simulink subsystem "soccer_ball_sub"  (R2022b)
settings: Solver=VariableStepAuto  StartTime=0.0  StopTime=10.0  RelTol=1e-3
settings Model: Creator=User  LastModifiedBy=ROG

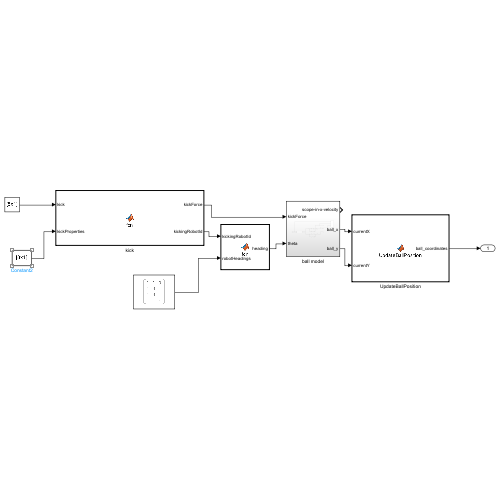
[thumbnail: Simulink's stored preview of the top-level diagram]
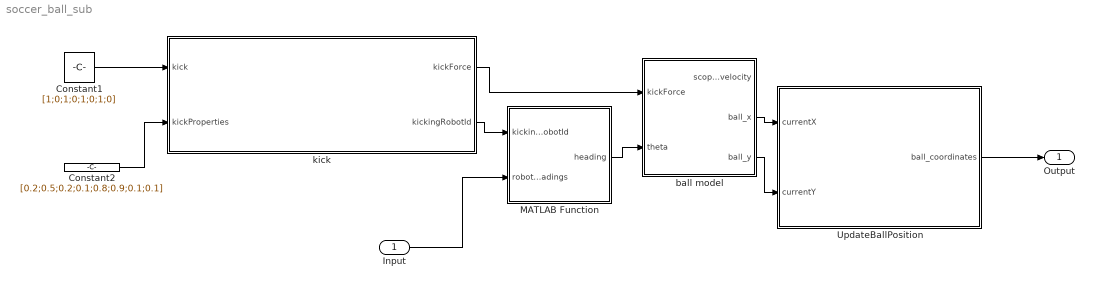
== system soccer_ball_sub ==
  Input : Inport
  Constant1 : Constant  Value=[1;0;1;0;1;0;1;0]
  Constant2 : Constant  Value=[0.2;0.5;0.2;0.1;0.8;0.9;0.1;0.1]
  MATLAB Function : MATLAB Function  TreatAsAtomicUnit=on
  UpdateBallPosition : MATLAB Function  TreatAsAtomicUnit=on
  ball model : Subsystem
  kick : MATLAB Function  TreatAsAtomicUnit=on
  Output : Outport
  wires:
  ball model/2(ball_x) -> UpdateBallPosition/1(currentX)
  kick/1(kickForce) -> ball model/1(kickForce)
  MATLAB Function/1(heading) -> ball model/2(theta)
  ball model/3(ball_y) -> UpdateBallPosition/2(currentY)
  UpdateBallPosition/1(ball_coordinates) -> Output/1
  kick/2(kickingRobotId) -> MATLAB Function/1(kickingRobotId)
  Input/1 -> MATLAB Function/2(robotHeadings)
  Constant1/1 -> kick/1(kick)
  Constant2/1 -> kick/2(kickProperties)

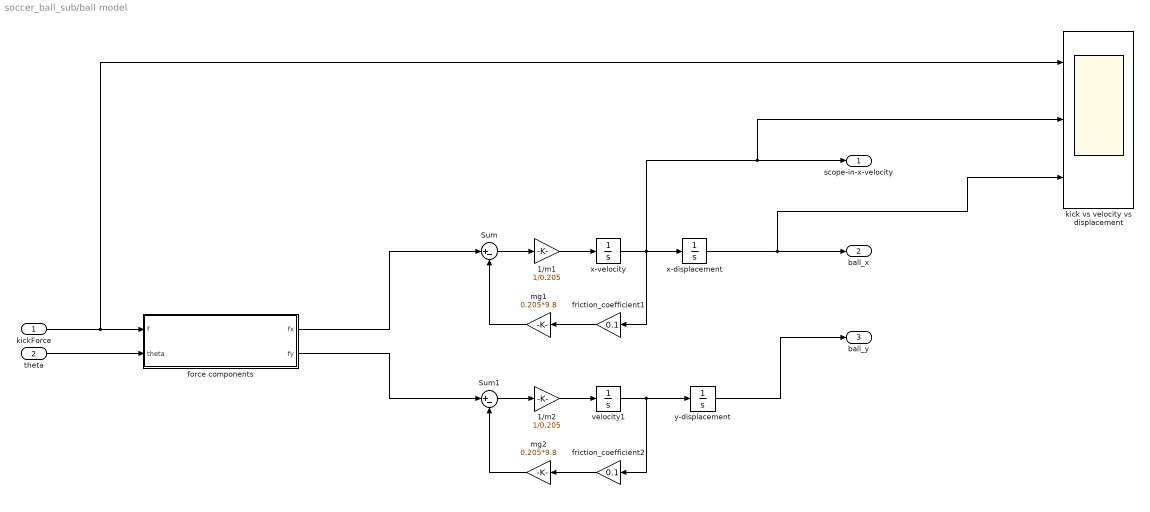
== system soccer_ball_sub/ball model ==
  kickForce : Inport
  theta : Inport  Port=2
  1/m1 : Gain  Gain=1/0.205
  1/m2 : Gain  Gain=1/0.205
  Sum : Sum  Inputs=|+-
  Sum1 : Sum  Inputs=|+-
  force components : MATLAB Function  TreatAsAtomicUnit=on
  friction_coefficient1 : Gain  Gain=0.1
  friction_coefficient2 : Gain  Gain=0.1
  kick vs velocity vs displacement : Scope  NumInputPorts=3
  mg1 : Gain  Gain=0.205*9.8
  mg2 : Gain  Gain=0.205*9.8
  velocity1 : Integrator
  x-displacement : Integrator
  x-velocity : Integrator
  y-displacement : Integrator
  scope-in-x-velocity : Outport
  ball_x : Outport  Port=2
  ball_y : Outport  Port=3
  wires:
  kickForce/1 -> force components/1(f), kick vs velocity vs displacement/1
  y-displacement/1 -> ball_y/1
  theta/1 -> force components/2(theta)
  x-displacement/1 -> ball_x/1, kick vs velocity vs displacement/3
  mg2/1 -> Sum1/2
  force components/1(fx) -> Sum/1
  1/m1/1 -> x-velocity/1
  Sum1/1 -> 1/m2/1
  force components/2(fy) -> Sum1/1
  friction_coefficient1/1 -> mg1/1
  1/m2/1 -> velocity1/1
  Sum/1 -> 1/m1/1
  mg1/1 -> Sum/2
  friction_coefficient2/1 -> mg2/1
  x-velocity/1 -> x-displacement/1, friction_coefficient1/1, scope-in-x-velocity/1, kick vs velocity vs displacement/2
  velocity1/1 -> y-displacement/1, friction_coefficient2/1

== matlab function soccer_ball_sub/UpdateBallPosition ==
  data: currentX input; ball_coordinates output; currentY input
function ball_coordinates  = UpdateBallPosition(currentX, currentY)

 
    % put heading in vector
    currentPosition = [currentX, currentY];
    
   
    % output the vector
    ball_coordinates = currentPosition;
end

== matlab function soccer_ball_sub/ball model/force components ==
  data: f input; fx output; theta input; fy output
function [fx,fy] = getForceComponents(f, theta)
    
    fx = f*cos((theta*pi)/180);
    fy = f*sin((theta*pi)/180);

end

== matlab function soccer_ball_sub/kick ==
  data: kickForce output; kick input; kickingRobotId output; kickProperties input
function [kickForce, kickingRobotId] = fcn(kick, kickProperties)

% kick id 8x1 matrix
% has boolean values of whether a robot kicks or not

kick_true = find(kick);

kickingRobotId = kick_true(randi(length(kick_true),1));

kickForce = kickProperties(kickingRobotId,1);

== matlab function soccer_ball_sub/MATLAB Function ==
  data: kickingRobotId input; heading output; robotHeadings input
function heading = fcn(kickingRobotId, robotHeadings)

heading = robotHeadings(kickingRobotId,1);
